simulink model "GLM1SIP_LQR_TORQUE17"  (R2015a)
settings: Solver=ode1  SolverMode=SingleTasking  StartTime=0.0  StopTime=inf  FixedStep=0.005  RelTol=1e-3
libraries: gtbox x6
settings Model: SimulationMode=external  ExtModeTrigDuration=200000  Creator=Administrator  LastModifiedBy=elec3200
settings DataIOCC: SignalLoggingSaveFormat=ModelDataLogs  SignalLoggingName=sigsOut
settings OptimizationCC: ExpressionDepthLimit=2147483647  InitFltsAndDblsToZero=on
settings DebuggingCC: SaveWithParameterizedLinksMsg=none  UnderspecifiedInitializationDetection=Classic  MergeDetectMultiDrivingBlocksExec=none  SignalResolutionControl=TryResolveAllWithWarning  MultiTaskDSMMsg=warning  MultiTaskCondExecSysMsg=none  FcnCallInpInsideContextMsg=UseLocalSettings  StateNameClashWarn=warning
settings HardwareCC: ProdBitPerLong=64  ProdBitPerPointer=64  ProdIntDivRoundTo=Zero  ProdEndianess=LittleEndian  ProdWordSize=64  ProdHWDeviceType=Intel->x86-64  TargetBitPerLong=64  TargetBitPerPointer=64  TargetIntDivRoundTo=Zero  TargetEndianess=LittleEndian  TargetWordSize=64  TargetHWDeviceType=Intel->x86-64
settings RTWCC: SystemTargetFile=rtwin.tlc  TemplateMakefile=rtwin.tmf  Description=Real-Time Windows Target
settings RTWinTargetCC: TargetFcnLib=ansi_tfl_tmw.mat  TargetPreCompLibLocation=C:\Program Files\MATLAB\R2015a\toolbox\sldrt\lib\win64  ModelReferenceCompliant=off  CompOptLevelCompliant=off

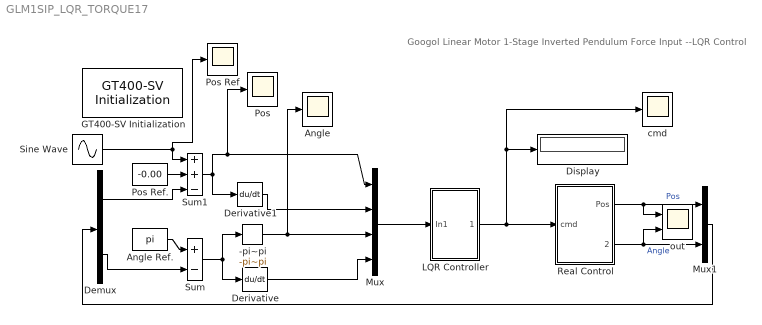
== system GLM1SIP_LQR_TORQUE17 ==
  note: Googol Linear Motor 1-Stage Inverted Pendulum
      | Force Input --LQR Control
  " -pi~pi" : gtbox/GT-400-SV Function Blocks/ -pi~pi
  Angle : Scope
      settings: TickLabels=on  TimeRange=200  YMin=-0.0175  YMax=0.0175  SaveName=Angle  MaxDataPoints=10000
  Angle Ref. : Constant  Value=pi
  Demux : Demux  Outputs=2
  Derivative : Derivative
  Derivative1 : Derivative
  Display : Display
  GT400-SV Initialization : gtbox/GT-400-SV Function Blocks/GT400-SV Initialization  Priority=0  openloop=1  comport=0
  LQR Controller : Subsystem  mask{x=-20, xdot=-13.6349, angle=38.7336, angledot=6.1233}
      mask prompts: x "Kx"; xdot "Kx'"; angle "Ka"; angledot "Ka'"
  Mux : Mux
  Mux1 : Mux  Inputs=2
  Pos : Scope
      settings: TickLabels=on  TimeRange=200  YMin=-0.045  YMax=0.035  SaveName=Pos  MaxDataPoints=10000
  Pos Ref : Scope
      settings: TimeRange=20  YMin=-0.1  YMax=0.1  SaveName=ScopeData2
  Pos Ref. : Constant  Value=-0.00
  Real Control : Subsystem
  Sine Wave : Sin  Amplitude=0.025  SampleTime=0
  Sum : Sum  Inputs=+-  SaturateOnIntegerOverflow=on
  Sum1 : Sum  Inputs=++-  SaturateOnIntegerOverflow=on
  cmd : Scope
      settings: TickLabels=on  TimeRange=200  YMin=-3.5  YMax=3.5  SaveName=Pos1  MaxDataPoints=10000
  out : Scope  NumInputPorts=2
      settings: TickLabels=on  TimeRange=20  YMin=-0.05~-3.155  YMax=0.05~-3.1275  SaveName=Pos2  MaxDataPoints=50000
  wires:
  Mux/1 -> LQR Controller/1(In1)
  Mux1/1 -> Demux/1
  Sum/1 -> " -pi~pi"/1, Derivative/1
  Derivative1/1 -> Mux/2
  Demux/2 -> Sum/2
  Derivative/1 -> Mux/4
  Sum1/1 -> Derivative1/1, Mux/1, Pos/1
  Real Control/2(Angle) -> out/2, Mux1/2  "Angle"
  Angle Ref./1 -> Sum/1
  " -pi~pi"/1 -> Mux/3, Angle/1
  Real Control/1(Pos) -> out/1, Mux1/1  "Pos"
  LQR Controller/1(Cmd) -> Display/1, cmd/1, Real Control/1(cmd)
  Demux/1 -> Sum1/3
  Pos Ref./1 -> Sum1/2
  Sine Wave/1 -> Pos Ref/1, Sum1/1

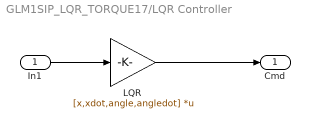
== system GLM1SIP_LQR_TORQUE17/LQR Controller ==
  In1 : Inport
  LQR : Gain  Gain=[x,xdot,angle,angledot]  Multiplication=Matrix(K*u)  SaturateOnIntegerOverflow=on  OutDataTypeStr=Inherit: Same as input  ParamDataTypeStr=Inherit: Same as input
  Cmd : Outport
  wires:
  In1/1 -> LQR/1
  LQR/1 -> Cmd/1

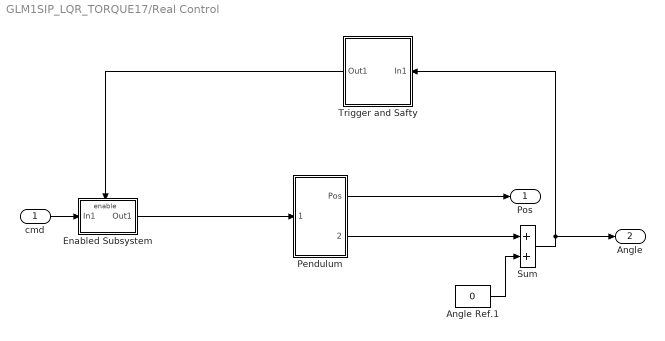
== system GLM1SIP_LQR_TORQUE17/Real Control ==
  cmd : Inport
  Angle Ref.1 : Constant  Value=0
  Enabled Subsystem : Subsystem  TreatAsAtomicUnit=on
  Pendulum : Subsystem
  Sum : Sum  SaturateOnIntegerOverflow=on
  Trigger and Safty : Subsystem
  Pos : Outport
  Angle : Outport  Port=2
  wires:
  Pendulum/1(Pos) -> Pos/1
  cmd/1 -> Enabled Subsystem/1(In1)
  Enabled Subsystem/1(Out1) -> Pendulum/1(Cmd)
  Trigger and Safty/1(Out1) -> Enabled Subsystem/Enable
  Pendulum/2(Angle) -> Sum/1
  Angle Ref.1/1 -> Sum/2
  Sum/1 -> Angle/1, Trigger and Safty/1(In1)

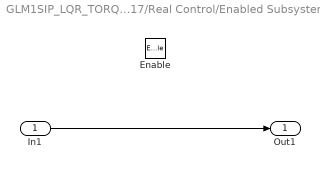
== system GLM1SIP_LQR_TORQUE17/Real Control/Enabled Subsystem ==
  In1 : Inport
  Enable : EnablePort
  Out1 : Outport
  wires:
  In1/1 -> Out1/1

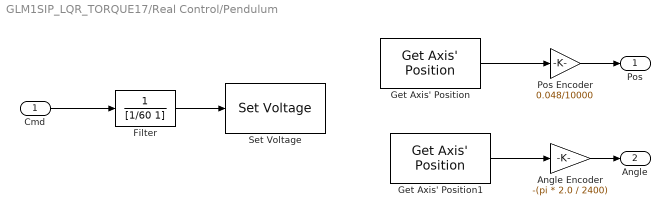
== system GLM1SIP_LQR_TORQUE17/Real Control/Pendulum ==
  Cmd : Inport
  Angle Encoder : Gain  Gain=-(pi * 2.0 / 2400)  SaturateOnIntegerOverflow=on  OutDataTypeStr=Inherit: Same as input  ParamDataTypeStr=Inherit: Same as input
  Filter : TransferFcn  Denominator=[1/60 1]
  Get Axis' Position : gtbox/GT-400-SV Function Blocks/Get Axis' Position  Priority=1  axis=1
  Get Axis' Position1 : gtbox/GT-400-SV Function Blocks/Get Axis' Position  Priority=1  axis=2
  Pos Encoder : Gain  Gain=0.048/10000  SaturateOnIntegerOverflow=on  OutDataTypeStr=Inherit: Same as input  ParamDataTypeStr=Inherit: Same as input
  Set Voltage : gtbox/GT-400-SV Function Blocks/Set Voltage  Priority=1  axis=1  back_cmd=1  back_pos=20000
  Pos : Outport
  Angle : Outport  Port=2
  wires:
  Angle Encoder/1 -> Angle/1
  Pos Encoder/1 -> Pos/1
  Get Axis' Position/1 -> Pos Encoder/1
  Cmd/1 -> Filter/1
  Get Axis' Position1/1 -> Angle Encoder/1
  Filter/1 -> Set Voltage/1

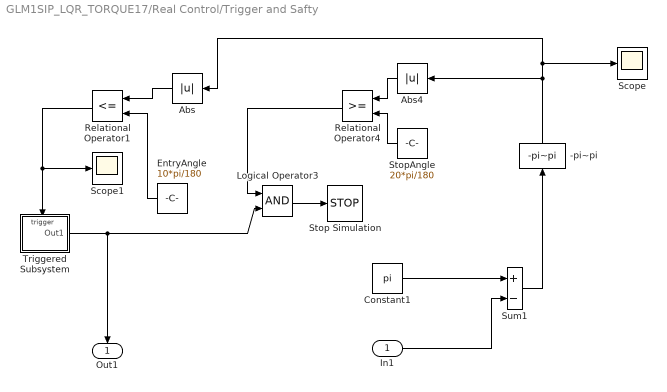
== system GLM1SIP_LQR_TORQUE17/Real Control/Trigger and Safty ==
  In1 : Inport
  " -pi~pi" : gtbox/GT-400-SV Function Blocks/ -pi~pi
  Abs : Abs  SaturateOnIntegerOverflow=on
  Abs4 : Abs  SaturateOnIntegerOverflow=on
  Constant1 : Constant  Value=pi
  EntryAngle : Constant  Value=10*pi/180
  Logical Operator3 : Logic  AllPortsSameDT=off
  Relational Operator1 : RelationalOperator  Operator=<=
  Relational Operator4 : RelationalOperator
  Scope : Scope
      settings: YMin=-3.134  YMax=-3.123
  Scope1 : Scope
      settings: YMin=-3.134  YMax=-3.123
  Stop Simulation : Stop
  StopAngle : Constant  Value=20*pi/180
  Sum1 : Sum  Inputs=+-  SaturateOnIntegerOverflow=on
  Triggered Subsystem : Subsystem  TreatAsAtomicUnit=on
  Out1 : Outport
  wires:
  Relational Operator4/1 -> Logical Operator3/1
  StopAngle/1 -> Relational Operator4/2
  Abs4/1 -> Relational Operator4/1
  Abs/1 -> Relational Operator1/1
  EntryAngle/1 -> Relational Operator1/2
  Relational Operator1/1 -> Scope1/1, Triggered Subsystem/Trigger
  Triggered Subsystem/1(Out1) -> Logical Operator3/2, Out1/1
  Logical Operator3/1 -> Stop Simulation/1
  " -pi~pi"/1 -> Abs4/1, Scope/1, Abs/1
  Constant1/1 -> Sum1/1
  In1/1 -> Sum1/2
  Sum1/1 -> " -pi~pi"/1

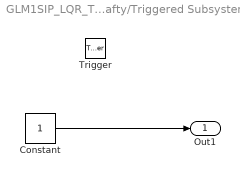
== system GLM1SIP_LQR_TORQUE17/Real Control/Trigger and Safty/Triggered Subsystem ==
  Trigger : TriggerPort
  Constant : Constant
  Out1 : Outport  InitialOutput=0
  wires:
  Constant/1 -> Out1/1
